simulink model "ahrs_filter"  (Simulink 7.7)
settings: Solver=ode45  StartTime=0.0  StopTime=30.0  RelTol=1e-3
settings Model: Creator=Korken  LastModifiedBy=Korken

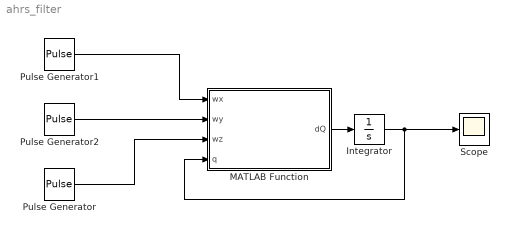
== system ahrs_filter ==
  Integrator : Integrator  InitialCondition=[1; 0; 0; 0]
  MATLAB Function : Stateflow chart  TreatAsAtomicUnit=on
  Pulse Generator : DiscretePulseGenerator  PulseType=Time based  Amplitude=0.03  Period=30  PulseWidth=33  PhaseDelay=20
  Pulse Generator1 : DiscretePulseGenerator  PulseType=Time based  Amplitude=0.03  Period=30  PulseWidth=33
  Pulse Generator2 : DiscretePulseGenerator  PulseType=Time based  Amplitude=0.03  Period=30  PulseWidth=33  PhaseDelay=10
  Scope : Scope
  wires:
  MATLAB Function/1(dQ) -> Integrator/1
  Pulse Generator1/1 -> MATLAB Function/1(wx)
  Pulse Generator2/1 -> MATLAB Function/2(wy)
  Integrator/1 -> MATLAB Function/4(q), Scope/1
  Pulse Generator/1 -> MATLAB Function/3(wz)

== matlab function MATLAB Function ==
  data: wx input double; dQ output double; wy input double; wz input double; q input double
function dQ = Quaternion_der(wx,wy,wz,q)
  w = -[wx;
       wy;
       wz];
   
  dQ2 = [-q(2), -q(3), -q(4);
        q(1), -q(4), q(3);
        q(4), q(1), -q(2);
        -q(3), q(2), q(1)]*w;
    
  dQ = [-q(2), -q(3), -q(4);
        q(1), q(4), -q(3);
        -q(4), q(1), q(2);
        q(3), -q(2), q(1)]*w;
    
end
